simulink model "simple_window"  (R2020a)
settings: Solver=FixedStepDiscrete  StartTime=0.0  StopTime=10.0  RelTol=1e-3
libraries: hdlsllib x5, simulink x2
settings Model: DataTypeOverride=Off  Creator=david  LastModifiedBy=david
settings OptimizationCC: BlockReduction=off  ConditionallyExecuteInputs=off  DefaultParameterBehavior=Inlined
settings DebuggingCC: AlgebraicLoopMsg=error  SingleTaskRateTransMsg=error
settings HardwareCC: ProdBitPerPointer=32  ProdBitPerSizeT=32  ProdBitPerPtrDiffT=32  ProdLargestAtomicFloat=None  ProdIntDivRoundTo=Undefined  ProdEndianess=Unspecified  ProdWordSize=32  ProdHWDeviceType=ASIC/FPGA->ASIC/FPGA  TargetBitPerPointer=64  TargetBitPerSizeT=64  TargetBitPerPtrDiffT=64  TargetLongLongMode=on  TargetIntDivRoundTo=Zero  TargetEndianess=LittleEndian  TargetWordSize=64  TargetHWDeviceType=Custom Processor->MATLAB Host Computer  ProdEqTarget=off

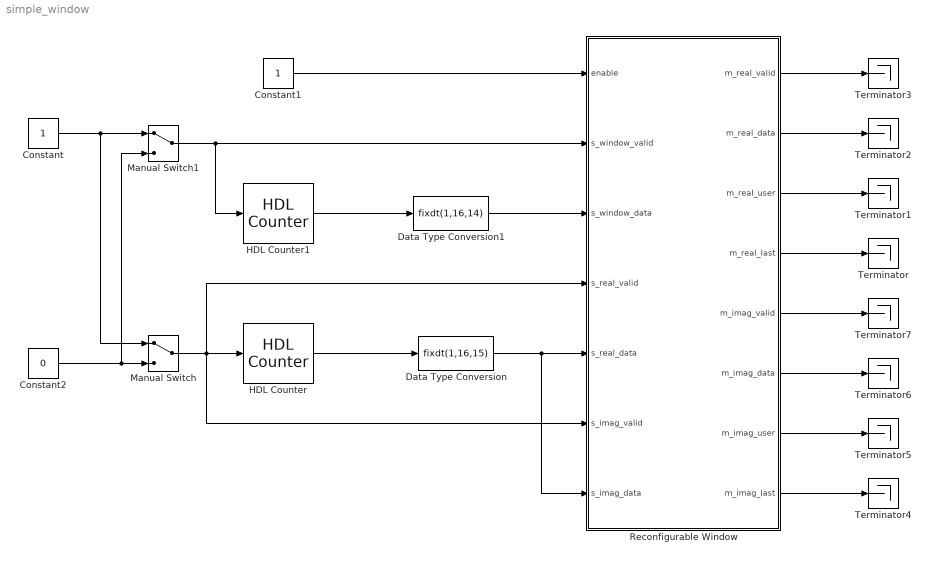
== system simple_window ==
  Constant : Constant  OutDataTypeStr=boolean  SampleTime=1/256e6
  Constant1 : Constant  OutDataTypeStr=boolean  SampleTime=1/256e6
  Constant2 : Constant  Value=0  OutDataTypeStr=boolean  SampleTime=1/256e6
  Data Type Conversion : DataTypeConversion  OutDataTypeStr=fixdt(1,16,15)  ConvertRealWorld=Stored Integer (SI)
  Data Type Conversion1 : DataTypeConversion  OutDataTypeStr=fixdt(1,16,14)  ConvertRealWorld=Stored Integer (SI)
  HDL Counter : hdlsllib/Sources/HDL Counter  CountType=Count limited  CountInit=0  CountStep=1  CountMax=2047  CountFromType=Initial value  CountFrom=0  CountResetPort=off  CountLoadPort=off  CountEnbPort=on  CountDirPort=off  CountDataType=Unsigned  CountWordLen=11  CountFracLen=0  CountSampTime=1
  HDL Counter1 : hdlsllib/Sources/HDL Counter  CountType=Count limited  CountInit=0  CountStep=1  CountMax=2047  CountFromType=Initial value  CountFrom=0  CountResetPort=off  CountLoadPort=off  CountEnbPort=on  CountDirPort=off  CountDataType=Unsigned  CountWordLen=11  CountFracLen=0  CountSampTime=1
  Manual Switch : ManualSwitch
  Manual Switch1 : ManualSwitch
  Reconfigurable Window : Subsystem  TreatAsAtomicUnit=on
  Terminator{,1..7} (8 alike) : Terminator
  wires:
  HDL Counter/1 -> Data Type Conversion/1
  Constant1/1 -> Reconfigurable Window/1(enable)
  Manual Switch/1 -> Reconfigurable Window/4(s_real_valid), Reconfigurable Window/6(s_imag_valid), HDL Counter/1
  Constant/1 -> Manual Switch/1, Manual Switch1/1
  Constant2/1 -> Manual Switch1/2, Manual Switch/2
  Reconfigurable Window/4(m_real_last) -> Terminator/1
  Reconfigurable Window/3(m_real_user) -> Terminator1/1
  Reconfigurable Window/2(m_real_data) -> Terminator2/1
  Reconfigurable Window/1(m_real_valid) -> Terminator3/1
  Data Type Conversion/1 -> Reconfigurable Window/7(s_imag_data), Reconfigurable Window/5(s_real_data)
  Manual Switch1/1 -> HDL Counter1/1, Reconfigurable Window/2(s_window_valid)
  HDL Counter1/1 -> Data Type Conversion1/1
  Reconfigurable Window/5(m_imag_valid) -> Terminator7/1
  Reconfigurable Window/6(m_imag_data) -> Terminator6/1
  Reconfigurable Window/7(m_imag_user) -> Terminator5/1
  Reconfigurable Window/8(m_imag_last) -> Terminator4/1
  Data Type Conversion1/1 -> Reconfigurable Window/3(s_window_data)

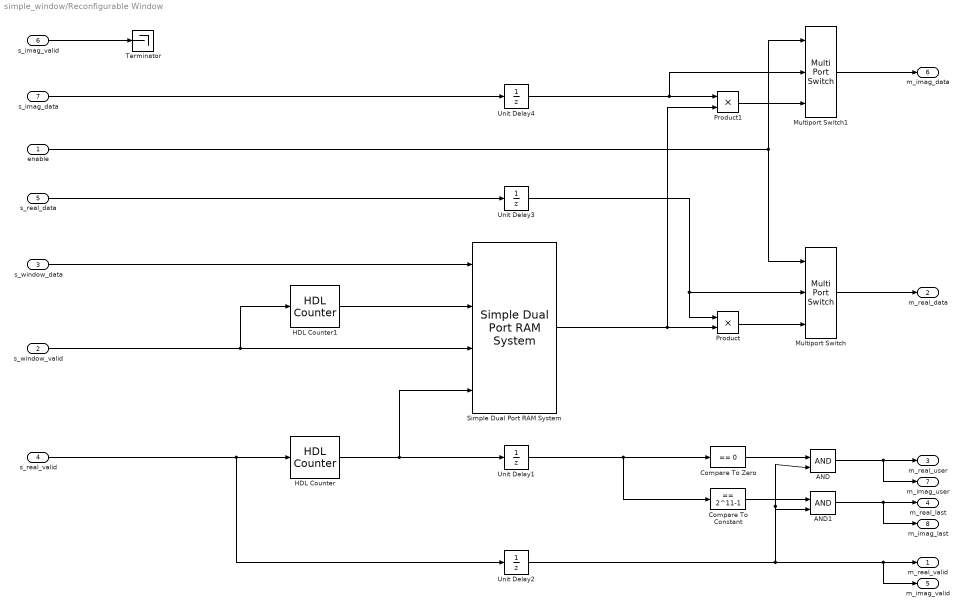
== system simple_window/Reconfigurable Window ==
  enable : Inport
  s_window_valid : Inport  Port=2
  s_window_data : Inport  Port=3
  s_real_valid : Inport  Port=4
  s_real_data : Inport  Port=5
  s_imag_valid : Inport  Port=6
  s_imag_data : Inport  Port=7
  AND : Logic  IconShape=distinctive  AllPortsSameDT=off  OutDataTypeStr=boolean
  AND1 : Logic  IconShape=distinctive  AllPortsSameDT=off  OutDataTypeStr=boolean
  Compare To Constant : simulink/Logic and Bit Operations/Compare To Constant  relop===  const=2^11-1  OutDataTypeStr=boolean
  Compare To Zero : simulink/Logic and Bit Operations/Compare To Zero  relop===  OutDataTypeStr=boolean
  HDL Counter : hdlsllib/Sources/HDL Counter  CountType=Count limited  CountInit=0  CountStep=1  CountMax=2^11-1  CountFromType=Initial value  CountFrom=0  CountResetPort=off  CountLoadPort=off  CountEnbPort=on  CountDirPort=off  CountDataType=Unsigned  CountWordLen=11  CountFracLen=0  CountSampTime=1
  HDL Counter1 : hdlsllib/Sources/HDL Counter  CountType=Count limited  CountInit=0  CountStep=1  CountMax=2^11-1  CountFromType=Initial value  CountFrom=0  CountResetPort=off  CountLoadPort=off  CountEnbPort=on  CountDirPort=off  CountDataType=Unsigned  CountWordLen=11  CountFracLen=0  CountSampTime=1
  Multiport Switch : MultiPortSwitch  DataPortOrder=Zero-based contiguous  Inputs=2  zeroidx=on
  Multiport Switch1 : MultiPortSwitch  DataPortOrder=Zero-based contiguous  Inputs=2  zeroidx=on
  Product : Product  OutDataTypeStr=Inherit: Same as first input
  Product1 : Product  OutDataTypeStr=Inherit: Same as first input
  Simple Dual Port RAM System : hdlsllib/HDL RAMs/Simple Dual Port RAM System  RAMType=Simple dual port  WriteOutputValue=New data  RAMInitialValue=[0:2^-11:1-2^-11]  SimulateUsing=Code generation
      settings: SourceProductBaseCode=SL
  Terminator : Terminator
  Unit Delay{1..4} (4 alike) : UnitDelay  SampleTime=-1  HasFrameUpgradeWarning=on
  m_real_valid : Outport
  m_real_data : Outport  Port=2
  m_real_user : Outport  Port=3
  m_real_last : Outport  Port=4
  m_imag_valid : Outport  Port=5
  m_imag_data : Outport  Port=6
  m_imag_user : Outport  Port=7
  m_imag_last : Outport  Port=8
  wires:
  s_window_valid/1 -> HDL Counter1/1, Simple Dual Port RAM System/3
  HDL Counter/1 -> Simple Dual Port RAM System/4, Unit Delay1/1
  HDL Counter1/1 -> Simple Dual Port RAM System/2
  s_real_valid/1 -> Unit Delay2/1, HDL Counter/1
  s_real_data/1 -> Unit Delay3/1
  Simple Dual Port RAM System/1 -> Product1/2, Product/2
  enable/1 -> Multiport Switch/1, Multiport Switch1/1
  Multiport Switch/1 -> m_real_data/1
  s_window_data/1 -> Simple Dual Port RAM System/1
  Product/1 -> Multiport Switch/3
  Unit Delay1/1 -> Compare To Constant/1, Compare To Zero/1
  Unit Delay2/1 -> AND/2, AND1/2, m_imag_valid/1, m_real_valid/1
  Unit Delay3/1 -> Multiport Switch/2, Product/1
  Compare To Zero/1 -> AND/1
  AND/1 -> m_imag_user/1, m_real_user/1
  Compare To Constant/1 -> AND1/1
  AND1/1 -> m_imag_last/1, m_real_last/1
  s_imag_data/1 -> Unit Delay4/1
  Product1/1 -> Multiport Switch1/3
  Unit Delay4/1 -> Multiport Switch1/2, Product1/1
  s_imag_valid/1 -> Terminator/1
  Multiport Switch1/1 -> m_imag_data/1
